simulink model "michelson_sim"  (R2019b)
settings: Solver=VariableStepAuto  StartTime=0.0  StopTime=10.0  RelTol=1e-3
settings Model: Creator=Vetter  LastModifiedBy=Vetter

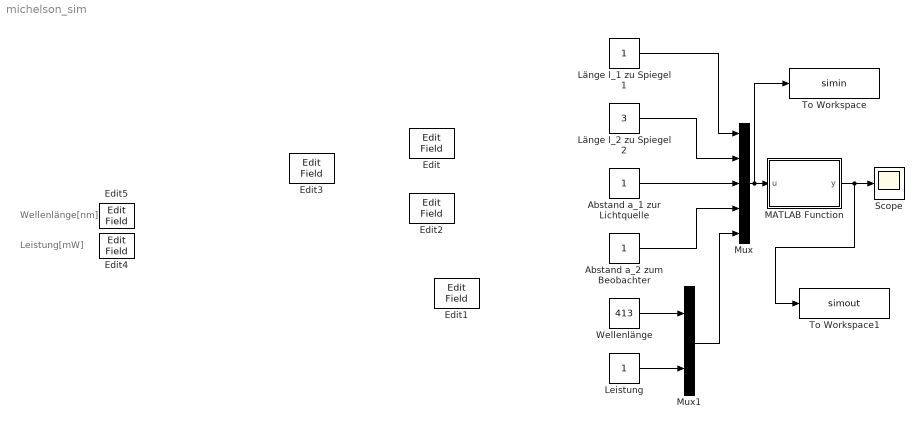
== system michelson_sim ==
  note: Wellenlänge[nm]
  note: Leistung[mW]
  Abstand a_1 zur Lichtquelle : Constant
  Abstand a_2 zum Beobachter : Constant
  Edit{,1..5} (6 alike) : EditField  LabelPosition=Hide  ShowInitialText=on  Alignment=Center
  Leistung : Constant
  "Länge l_1 zu Spiegel 1 " : Constant
  "Länge l_2 zu Spiegel 2 " : Constant  Value=3
  MATLAB Function : MATLAB Function  TreatAsAtomicUnit=on
  Mux : Mux  Inputs=5
  Mux1 : Mux  Inputs=2
  Scope : Scope
  To Workspace : ToWorkspace  VariableName=simin  SaveFormat=Timeseries  SampleTime=-1
  To Workspace1 : ToWorkspace  VariableName=simout  SaveFormat=Timeseries  SampleTime=-1
  "Wellenlänge " : Constant  Value=413
  wires:
  MATLAB Function/1(y) -> To Workspace1/1, Scope/1
  Mux/1 -> To Workspace/1, MATLAB Function/1(u)
  "Länge l_1 zu Spiegel 1 "/1 -> Mux/1
  "Länge l_2 zu Spiegel 2 "/1 -> Mux/2
  Abstand a_1 zur Lichtquelle/1 -> Mux/3
  Abstand a_2 zum Beobachter/1 -> Mux/4
  Mux1/1 -> Mux/5
  "Wellenlänge "/1 -> Mux1/1
  Leistung/1 -> Mux1/2

== matlab function michelson_sim/MATLAB Function ==
  data: u input; y output
function y = michelson(u)

% Konstanten
c = 299792458;
d_const = 8.854187817*10^(-12);

% Funktionsparameter mit Umrechnung in SI-Einheiten
l_1 = u(1);
l_2 = u(2);
a_1 = u(3); 
a_2 = u(4); 
wellenlaenge = u(5)*10^(-9); 
leistung = u(6)*10^(-3); 

%Berechnung der Lichtquellenamplitude E_0 
E_0 = sqrt(2*(leistung)/(c*d_const));

%Berechnung der Periodendauer 
T = wellenlaenge/c;

%Berechnung des Betrages des Wellenvektors
k = 2*pi/wellenlaenge; 

%Berechnung der Eigenkreisfrequenz
w = 2*pi/T; 
z = 1; 
syms t;

E_1 = E_0*exp(i*(k*z-w*t));
E_2 = E_0*exp(i*(k*z-w*t));



E_ges = E_1 + E_2


y = u;
